simulink model "lab13try1_2024a"  (R2024a)
settings: Solver=VariableStepAuto  StartTime=0.0  StopTime=250  RelTol=1e-3  EnableMultiTasking=on
values from neighbouring files (symbols this model uses):
  CDdatum = CD(1:47,2)    [Presimulink.m]
  CLdatum = CL(1:47,2)    [Presimulink.m]
  Cmdatum = Cm(1:47,2)    [Presimulink.m]
  dCDelev = [dCDn10 dCDn5 dCD0 dCDp5 dCDp10]    [Presimulink.m]
  dCLelev = [dCLn10 dCLn5 dCL0 dCLp5 dCLp10]    [Presimulink.m]
  dCmelev = [dCmn10 dCmn5 dCm0 dCmp5 dCmp10]    [Presimulink.m]
undefined symbols (not defined in the file or in its folder): Cn_datum, Croll_datum, CY_datum, dCn_aileron, dCn_rudder, dCroll_aileron, dCroll_rudder, dCY_aileron, dCY_rudder
libraries: aerolibconvert2 x6, slpidlib x4, aerolibasang x2, shared6dof x1, aerolibadyn x1, aerolibanim x1
settings Model: Creator=davidrwilliams  LastModifiedBy=xan2
settings SolverCC: AlgebraicLoopSolver=TrustRegion
settings DataIOCC: LimitDataPoints=on  ReturnWorkspaceOutputs=off
settings OptimizationCC: ReuseModelBlockBuffer=off  LifeSpan=inf
settings DebuggingCC: UnconnectedInputMsg=warning  UnconnectedOutputMsg=warning  UnconnectedLineMsg=warning  AllowSymbolicDim=off  SFUnexpectedBacktrackingDiag=warning  SFNoUnconditionalDefaultTransitionDiag=warning  SFExecutionAtInitializationDiag=none  ArithmeticOperatorsInVariantConditions=warning
settings ModelReferenceCC: EnableRefExpFcnMdlSchedulingChecks=on  PropagateSignalLabelsOutOfModel=off
settings SFSimCC: SimUseLocalCustomCode=off  CustomCodeUndefinedFunction=UseInterfaceOnly
settings RTWCC: RTWUseLocalCustomCode=off  GPUComputeCapability=3.5
settings CodeAppCC: StateflowObjectComments=on
settings GRTTargetCC: TargetLangStandard=C89/C90 (ANSI)
settings ConfigComp: CovMetricSettings=dw  CovSaveCumulativeToWorkspaceVar=on  CovSaveSingleToWorkspaceVar=on  CovExternalEMLEnable=off  CovBoundaryAbsTol=1.0e-5

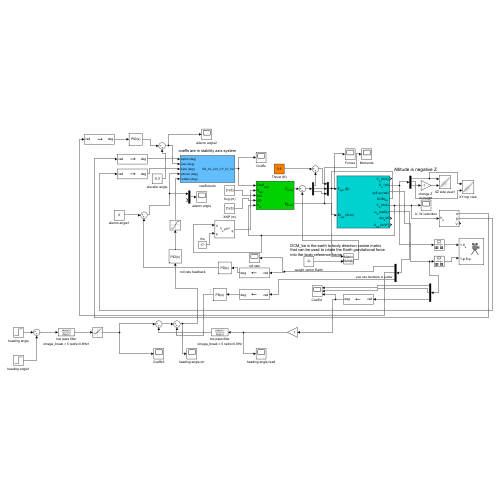
[thumbnail: Simulink's stored preview of the top-level diagram]
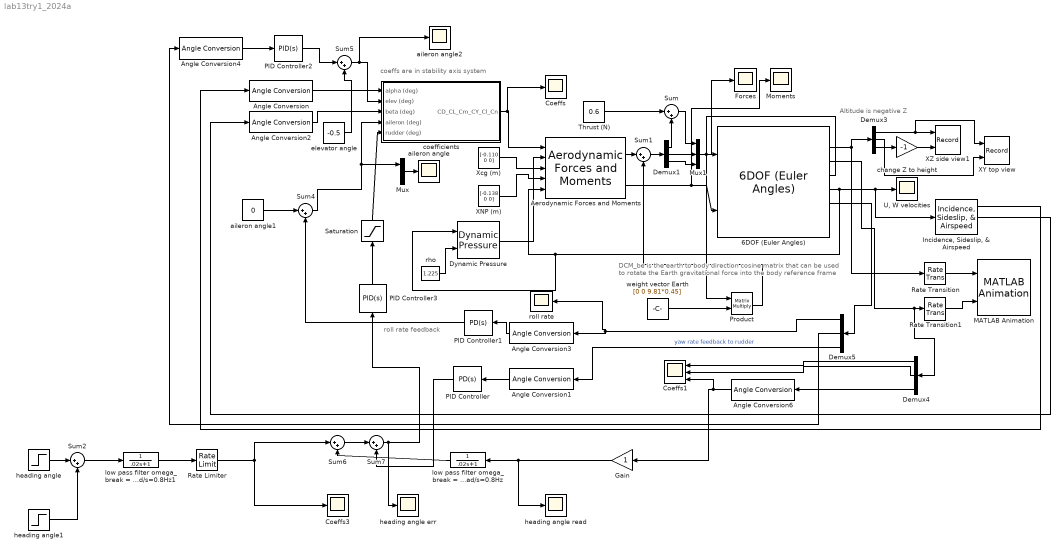
== system lab13try1_2024a ==
  note: roll rate feedback
  note: DCM_be is the earth to body direction cosine matrix
      | that can be used to rotate the Earth gravitational force
      | into the body reference frame
  note: Altitude is negative Z
  note: coeffs are in stability axis system
  6DOF (Euler Angles) : shared6dof/6DOF (Euler Angles)  units=Metric (MKS)  mtype=Fixed  rep=Euler Angles  xme_0=[0 0 -200]  Vm_0=[15 0 2.5]  eul_0=[0 1.4*pi/180 0]  pm_0=[0 0 0]  mass_0=0.45  mass_e=0.5  mass_f=2.0  inertia=[0.00083 0. -0.00118; 0. 0.0428 0.0; -0.00118 0.0 0.0433]  inertia_e=eye(3)  inertia_f=2*eye(3)  k_quat=1.0  vre_flag=on  abi_flag=off  aMode=aMode  xme_statename=''  Vm_statename=''  eul_statename=''  quat_statename=''  pm_statename=''  mass_statename=''
  "Aerodynamic Forces and Moments " : aerolibadyn/Aerodynamic Forces and Moments   inputAxes=Stability  outputForceAxes=Body  outputMomentAxes=Body  S=0.15  b=1  cbar=0.156
  Angle Conversion{,1..4,6} (6 alike) : aerolibconvert2/Angle Conversion  IU=rad  OU=deg
  Coeffs : Scope
  Coeffs1 : Scope  NumInputPorts=3
  Coeffs3 : Scope
  Demux{1,3..5} (4 alike) : Demux  Outputs=3
  Dynamic Pressure : aerolibasang/Dynamic Pressure
  Forces : Scope
  Gain : Gain
  "Incidence, Sideslip, & Airspeed" : aerolibasang/Incidence, Sideslip, & Airspeed
  MATLAB Animation : aerolibanim/MATLAB Animation  Tag=Matlab Animation 6 DOF  Vehicles=1  Geometries='astredwedge.mat'  BoundingBoxCoordinates=[-50,50,-50,50,-50,50]  CameraOffset=[-150,-50,0]  CameraViewAngle=3  SampleTime=0.2  FigurePosition=[8.014000e+02,2.082000e+02,4.480000e+02,3.540000e+02]
  Moments : Scope
  Mux : Mux  Inputs=2
  Mux1 : Mux  Inputs=3
  PID Controller : slpidlib/PID Controller  Controller=PD  Form=Parallel  TimeDomain=Continuous-time  UseExternalTs=off  SampleTime=-1  IntegratorMethod=Forward Euler  FilterMethod=Forward Euler  ControllerParametersSource=internal  P=0.005  I=1  UseKiTs=off  D=0  UseExternalDerivativeSource=off  N=100  UseFilter=on  TunerSelectOption=Transfer Function Based (PID Tuner App)  InitialConditionSource=internal  InitialConditionForIntegrator=0  InitialConditionForFilter=0  DifferentiatorICPrevScaledInput=0  ExternalReset=none  TrackingMode=off  Kt=1  LimitOutput=off  SatLimitsSource=internal  UpperSaturationLimit=inf  LowerSaturationLimit=-inf  LinearizeAsGain=on  AntiWindupMode=none  Kb=1  LimitIntegrator=off  UpperIntegratorSaturationLimit=inf  LowerIntegratorSaturationLimit=-inf  POutMin=[]  POutMax=[]  IOutMin=[]  IOutMax=[]  DOutMin=[]  DOutMax=[]  NOutMin=[]  NOutMax=[]  SumOutMin=[]  SumOutMax=[]  SaturationOutMin=[]  SaturationOutMax=[]  PParamMin=[]  PParamMax=[]  IParamMin=[]  IParamMax=[]  DParamMin=[]  DParamMax=[]  NParamMin=[]  NParamMax=[]  KbParamMin=[]  KbParamMax=[]  KtParamMin=[]  KtParamMax=[]  KbOutMin=[]  KbOutMax=[]  KtOutMin=[]  KtOutMax=[]  IntegratorOutMin=[]  IntegratorOutMax=[]  FilterOutMin=[]  FilterOutMax=[]  SumI1OutMin=[]  SumI1OutMax=[]  SumI2OutMin=[]  SumI2OutMax=[]  SumI3OutMin=[]  SumI3OutMax=[]  SumI4OutMin=[]  SumI4OutMax=[]  SumDOutMin=[]  SumDOutMax=[]  DifferentiatorOutMin=[]  DifferentiatorOutMax=[]  FilterDiffOutCoefMin=[]  FilterDiffOutCoefMax=[]  ReciprocalOutMin=[]  ReciprocalOutMax=[]  SumDenOutMin=[]  SumDenOutMax=[]  SumNumOutMin=[]  SumNumOutMax=[]  DivideOutMin=[]  DivideOutMax=[]  UdiffTsProdOutMin=[]  UdiffTsProdOutMax=[]  NTsProdOutMin=[]  NTsProdOutMax=[]  UintegralTsProdOutMin=[]  UintegralTsProdOutMax=[]  UngainTsProdOutMin=[]  UngainTsProdOutMax=[]  ClampingZeroOutDataTypeStr=Inherit: Inherit via back propagation  ClampingZeroOutMin=[]  ClampingZeroOutMax=[]  FilterDenConstantOutDataTypeStr=Inherit: Inherit via back propagation  FilterDenConstantOutMin=[]  FilterDenConstantOutMax=[]  PCopyOutDataTypeStr=Inherit: Inherit via back propagation  PCopyOutMin=[]  PCopyOutMax=[]  NCopyOutDataTypeStr=Inherit: Inherit via back propagation  NCopyOutMin=[]  NCopyOutMax=[]  IntegratorContinuousStateAttributes=''  IntegratorStateMustResolveToSignalObject=off  IntegratorRTWStateStorageClass=Auto  FilterContinuousStateAttributes=''  FilterStateMustResolveToSignalObject=off  FilterRTWStateStorageClass=Auto  ParallelPVariant=InternalParameters  IdealPVariant=Disabled  IVariant=Disabled  DVariant=InternalParameters  IntegratorVariant=Disabled  SatVariant=Disabled  AWVariant=Disabled  PCopyVariant=Disabled  TRVariant=Disabled  FdbkBlocksVariant=Forward  IdealPFdbkVariant=Disabled  SatFdbkVariant=Disabled  DerivativeFilterVariant=ContFilter  NVariant=InternalParameters  NCopyVariant=Disabled  FilterICVariant=InternalICsFilter  IntegratorICVariant=Disabled  ExternalResetVariant=Disabled  TRSumVariant=Passthrough  SumFdbkVariant=Disabled  SumVariant=Sum_PD  TsampFilterVariant=InternalTs  TsampNgainVariant=Passthrough  TsampIntegralVariant=Disabled_SignalSpec  ExternalSaturationOutDataTypeStr=Inherit: Same as second input  DerivativeSourceVariant=ErrorSignal
  PID Controller1 : slpidlib/PID Controller  Controller=PD  Form=Parallel  TimeDomain=Continuous-time  UseExternalTs=off  SampleTime=-1  IntegratorMethod=Forward Euler  FilterMethod=Forward Euler  ControllerParametersSource=internal  P=-0.5  I=1  UseKiTs=off  D=0  UseExternalDerivativeSource=off  N=100  UseFilter=on  TunerSelectOption=Transfer Function Based (PID Tuner App)  InitialConditionSource=internal  InitialConditionForIntegrator=0  InitialConditionForFilter=0  DifferentiatorICPrevScaledInput=0  ExternalReset=none  TrackingMode=off  Kt=1  LimitOutput=off  SatLimitsSource=internal  UpperSaturationLimit=inf  LowerSaturationLimit=-inf  LinearizeAsGain=on  AntiWindupMode=none  Kb=1  LimitIntegrator=off  UpperIntegratorSaturationLimit=inf  LowerIntegratorSaturationLimit=-inf  POutMin=[]  POutMax=[]  IOutMin=[]  IOutMax=[]  DOutMin=[]  DOutMax=[]  NOutMin=[]  NOutMax=[]  SumOutMin=[]  SumOutMax=[]  SaturationOutMin=[]  SaturationOutMax=[]  PParamMin=[]  PParamMax=[]  IParamMin=[]  IParamMax=[]  DParamMin=[]  DParamMax=[]  NParamMin=[]  NParamMax=[]  KbParamMin=[]  KbParamMax=[]  KtParamMin=[]  KtParamMax=[]  KbOutMin=[]  KbOutMax=[]  KtOutMin=[]  KtOutMax=[]  IntegratorOutMin=[]  IntegratorOutMax=[]  FilterOutMin=[]  FilterOutMax=[]  SumI1OutMin=[]  SumI1OutMax=[]  SumI2OutMin=[]  SumI2OutMax=[]  SumI3OutMin=[]  SumI3OutMax=[]  SumI4OutMin=[]  SumI4OutMax=[]  SumDOutMin=[]  SumDOutMax=[]  DifferentiatorOutMin=[]  DifferentiatorOutMax=[]  FilterDiffOutCoefMin=[]  FilterDiffOutCoefMax=[]  ReciprocalOutMin=[]  ReciprocalOutMax=[]  SumDenOutMin=[]  SumDenOutMax=[]  SumNumOutMin=[]  SumNumOutMax=[]  DivideOutMin=[]  DivideOutMax=[]  UdiffTsProdOutMin=[]  UdiffTsProdOutMax=[]  NTsProdOutMin=[]  NTsProdOutMax=[]  UintegralTsProdOutMin=[]  UintegralTsProdOutMax=[]  UngainTsProdOutMin=[]  UngainTsProdOutMax=[]  ClampingZeroOutDataTypeStr=Inherit: Inherit via back propagation  ClampingZeroOutMin=[]  ClampingZeroOutMax=[]  FilterDenConstantOutDataTypeStr=Inherit: Inherit via back propagation  FilterDenConstantOutMin=[]  FilterDenConstantOutMax=[]  PCopyOutDataTypeStr=Inherit: Inherit via back propagation  PCopyOutMin=[]  PCopyOutMax=[]  NCopyOutDataTypeStr=Inherit: Inherit via back propagation  NCopyOutMin=[]  NCopyOutMax=[]  IntegratorContinuousStateAttributes=''  IntegratorStateMustResolveToSignalObject=off  IntegratorRTWStateStorageClass=Auto  FilterContinuousStateAttributes=''  FilterStateMustResolveToSignalObject=off  FilterRTWStateStorageClass=Auto  ParallelPVariant=InternalParameters  IdealPVariant=Disabled  IVariant=Disabled  DVariant=InternalParameters  IntegratorVariant=Disabled  SatVariant=Disabled  AWVariant=Disabled  PCopyVariant=Disabled  TRVariant=Disabled  FdbkBlocksVariant=Forward  IdealPFdbkVariant=Disabled  SatFdbkVariant=Disabled  DerivativeFilterVariant=ContFilter  NVariant=InternalParameters  NCopyVariant=Disabled  FilterICVariant=InternalICsFilter  IntegratorICVariant=Disabled  ExternalResetVariant=Disabled  TRSumVariant=Passthrough  SumFdbkVariant=Disabled  SumVariant=Sum_PD  TsampFilterVariant=InternalTs  TsampNgainVariant=Passthrough  TsampIntegralVariant=Disabled_SignalSpec  ExternalSaturationOutDataTypeStr=Inherit: Same as second input  DerivativeSourceVariant=ErrorSignal
  PID Controller2 : slpidlib/PID Controller  Controller=PID  Form=Parallel  TimeDomain=Continuous-time  UseExternalTs=off  SampleTime=-1  IntegratorMethod=Forward Euler  FilterMethod=Forward Euler  ControllerParametersSource=internal  P=1  I=0  UseKiTs=off  D=0  UseExternalDerivativeSource=off  N=100  UseFilter=on  TunerSelectOption=Transfer Function Based (PID Tuner App)  InitialConditionSource=internal  InitialConditionForIntegrator=0  InitialConditionForFilter=0  DifferentiatorICPrevScaledInput=0  ExternalReset=none  TrackingMode=off  Kt=1  LimitOutput=off  SatLimitsSource=internal  UpperSaturationLimit=inf  LowerSaturationLimit=-inf  LinearizeAsGain=on  AntiWindupMode=none  Kb=1  LimitIntegrator=off  UpperIntegratorSaturationLimit=inf  LowerIntegratorSaturationLimit=-inf  POutMin=[]  POutMax=[]  IOutMin=[]  IOutMax=[]  DOutMin=[]  DOutMax=[]  NOutMin=[]  NOutMax=[]  SumOutMin=[]  SumOutMax=[]  SaturationOutMin=[]  SaturationOutMax=[]  PParamMin=[]  PParamMax=[]  IParamMin=[]  IParamMax=[]  DParamMin=[]  DParamMax=[]  NParamMin=[]  NParamMax=[]  KbParamMin=[]  KbParamMax=[]  KtParamMin=[]  KtParamMax=[]  KbOutMin=[]  KbOutMax=[]  KtOutMin=[]  KtOutMax=[]  IntegratorOutMin=[]  IntegratorOutMax=[]  FilterOutMin=[]  FilterOutMax=[]  SumI1OutMin=[]  SumI1OutMax=[]  SumI2OutMin=[]  SumI2OutMax=[]  SumI3OutMin=[]  SumI3OutMax=[]  SumI4OutMin=[]  SumI4OutMax=[]  SumDOutMin=[]  SumDOutMax=[]  DifferentiatorOutMin=[]  DifferentiatorOutMax=[]  FilterDiffOutCoefMin=[]  FilterDiffOutCoefMax=[]  ReciprocalOutMin=[]  ReciprocalOutMax=[]  SumDenOutMin=[]  SumDenOutMax=[]  SumNumOutMin=[]  SumNumOutMax=[]  DivideOutMin=[]  DivideOutMax=[]  UdiffTsProdOutMin=[]  UdiffTsProdOutMax=[]  NTsProdOutMin=[]  NTsProdOutMax=[]  UintegralTsProdOutMin=[]  UintegralTsProdOutMax=[]  UngainTsProdOutMin=[]  UngainTsProdOutMax=[]  ClampingZeroOutDataTypeStr=Inherit: Inherit via back propagation  ClampingZeroOutMin=[]  ClampingZeroOutMax=[]  FilterDenConstantOutDataTypeStr=Inherit: Inherit via back propagation  FilterDenConstantOutMin=[]  FilterDenConstantOutMax=[]  PCopyOutDataTypeStr=Inherit: Inherit via back propagation  PCopyOutMin=[]  PCopyOutMax=[]  NCopyOutDataTypeStr=Inherit: Inherit via back propagation  NCopyOutMin=[]  NCopyOutMax=[]  IntegratorContinuousStateAttributes=''  IntegratorStateMustResolveToSignalObject=off  IntegratorRTWStateStorageClass=Auto  FilterContinuousStateAttributes=''  FilterStateMustResolveToSignalObject=off  FilterRTWStateStorageClass=Auto  ParallelPVariant=InternalParameters  IdealPVariant=Disabled  IVariant=InternalParameters  DVariant=InternalParameters  IntegratorVariant=Continuous  SatVariant=Disabled  AWVariant=Passthrough  PCopyVariant=Disabled  TRVariant=Disabled  FdbkBlocksVariant=Forward  IdealPFdbkVariant=Disabled  SatFdbkVariant=Disabled  DerivativeFilterVariant=ContFilter  NVariant=InternalParameters  NCopyVariant=Disabled  FilterICVariant=InternalICsFilter  IntegratorICVariant=InternalICs  ExternalResetVariant=Disabled  TRSumVariant=Passthrough  SumFdbkVariant=Disabled  SumVariant=Sum_PID  TsampFilterVariant=InternalTs  TsampNgainVariant=Passthrough  TsampIntegralVariant=Disabled_SignalSpec  ExternalSaturationOutDataTypeStr=Inherit: Same as second input  DerivativeSourceVariant=ErrorSignal
  PID Controller3 : slpidlib/PID Controller  Controller=PID  Form=Parallel  TimeDomain=Continuous-time  UseExternalTs=off  SampleTime=-1  IntegratorMethod=Forward Euler  FilterMethod=Forward Euler  ControllerParametersSource=internal  P=1  I=0  UseKiTs=off  D=0.3  UseExternalDerivativeSource=off  N=100  UseFilter=on  TunerSelectOption=Transfer Function Based (PID Tuner App)  InitialConditionSource=internal  InitialConditionForIntegrator=0  InitialConditionForFilter=0  DifferentiatorICPrevScaledInput=0  ExternalReset=none  TrackingMode=off  Kt=1  LimitOutput=off  SatLimitsSource=internal  UpperSaturationLimit=inf  LowerSaturationLimit=-inf  LinearizeAsGain=on  AntiWindupMode=none  Kb=1  LimitIntegrator=off  UpperIntegratorSaturationLimit=inf  LowerIntegratorSaturationLimit=-inf  POutMin=[]  POutMax=[]  IOutMin=[]  IOutMax=[]  DOutMin=[]  DOutMax=[]  NOutMin=[]  NOutMax=[]  SumOutMin=[]  SumOutMax=[]  SaturationOutMin=[]  SaturationOutMax=[]  PParamMin=[]  PParamMax=[]  IParamMin=[]  IParamMax=[]  DParamMin=[]  DParamMax=[]  NParamMin=[]  NParamMax=[]  KbParamMin=[]  KbParamMax=[]  KtParamMin=[]  KtParamMax=[]  KbOutMin=[]  KbOutMax=[]  KtOutMin=[]  KtOutMax=[]  IntegratorOutMin=[]  IntegratorOutMax=[]  FilterOutMin=[]  FilterOutMax=[]  SumI1OutMin=[]  SumI1OutMax=[]  SumI2OutMin=[]  SumI2OutMax=[]  SumI3OutMin=[]  SumI3OutMax=[]  SumI4OutMin=[]  SumI4OutMax=[]  SumDOutMin=[]  SumDOutMax=[]  DifferentiatorOutMin=[]  DifferentiatorOutMax=[]  FilterDiffOutCoefMin=[]  FilterDiffOutCoefMax=[]  ReciprocalOutMin=[]  ReciprocalOutMax=[]  SumDenOutMin=[]  SumDenOutMax=[]  SumNumOutMin=[]  SumNumOutMax=[]  DivideOutMin=[]  DivideOutMax=[]  UdiffTsProdOutMin=[]  UdiffTsProdOutMax=[]  NTsProdOutMin=[]  NTsProdOutMax=[]  UintegralTsProdOutMin=[]  UintegralTsProdOutMax=[]  UngainTsProdOutMin=[]  UngainTsProdOutMax=[]  ClampingZeroOutDataTypeStr=Inherit: Inherit via back propagation  ClampingZeroOutMin=[]  ClampingZeroOutMax=[]  FilterDenConstantOutDataTypeStr=Inherit: Inherit via back propagation  FilterDenConstantOutMin=[]  FilterDenConstantOutMax=[]  PCopyOutDataTypeStr=Inherit: Inherit via back propagation  PCopyOutMin=[]  PCopyOutMax=[]  NCopyOutDataTypeStr=Inherit: Inherit via back propagation  NCopyOutMin=[]  NCopyOutMax=[]  IntegratorContinuousStateAttributes=''  IntegratorStateMustResolveToSignalObject=off  IntegratorRTWStateStorageClass=Auto  FilterContinuousStateAttributes=''  FilterStateMustResolveToSignalObject=off  FilterRTWStateStorageClass=Auto  ParallelPVariant=InternalParameters  IdealPVariant=Disabled  IVariant=InternalParameters  DVariant=InternalParameters  IntegratorVariant=Continuous  SatVariant=Disabled  AWVariant=Passthrough  PCopyVariant=Disabled  TRVariant=Disabled  FdbkBlocksVariant=Forward  IdealPFdbkVariant=Disabled  SatFdbkVariant=Disabled  DerivativeFilterVariant=ContFilter  NVariant=InternalParameters  NCopyVariant=Disabled  FilterICVariant=InternalICsFilter  IntegratorICVariant=InternalICs  ExternalResetVariant=Disabled  TRSumVariant=Passthrough  SumFdbkVariant=Disabled  SumVariant=Sum_PID  TsampFilterVariant=InternalTs  TsampNgainVariant=Passthrough  TsampIntegralVariant=Disabled_SignalSpec  ExternalSaturationOutDataTypeStr=Inherit: Same as second input  DerivativeSourceVariant=ErrorSignal
  Product : Product  Multiplication=Matrix(*)
  Rate Limiter : RateLimiter  RisingSlewLimit=10  FallingSlewLimit=-10  SampleTimeMode=inherited
  Rate Transition : RateTransition
  Rate Transition1 : RateTransition
  Saturation : Saturate  UpperLimit=10  LowerLimit=-10
  Sum{,1..2,4..7} (7 alike) : Sum  Inputs=|++
  Thrust (N) : Constant  Value=0.6
  "U, W velocities" : Scope
  XNP (m) : Constant  Value=[-0.138 0 0]
  XY top view : Record  FileSettingsInternal="{\"entries\":[{\"content\":{\"excelSettings\":{\"content\":{},\"type\":\"Streamout.ExcelSettings\"},\"parquetSettings\":{\"content\":{},\"type\":\"Streamout.ParquetSettings\"}},\"type\":\"Streamout.FileSettingStorage\",\"uuid\":\"\"}],\"packageUris\":[\"http:\\/\\/schema.mathworks.com\\/mf0\\/streamout_blocks\\/R2020a\"],\"version\":\"1.0\"}"  Layout=[1 1]  SignalsInternal="{\"entries\":[{\"content\":{\"signals\":[{\"content\":{\"blockPath\":[],\"dimensions\":[1],\"domain\":\"\",\"lineColor\":\"#a2142f\",\"plots\":[ 1 ],\"port\":1,\"signalID\":1,\"signalName\":\"Demux3:1\"},\"type\":\"RecordBlkView.Signal\",\"uuid\":\"\"},{\"content\":{\"blockPath\":[],\"dimensions\":[1],\"domain\":\"\",\"lineColor\":\"#139fff\",\"plots\":[ 1 ],\"port\":2,\"signalID\":2,\"signalName\":\"Demux3:2\"},\"type\":\"RecordBlkView.Signal\",\"uuid\":\"\"}]},\"type\":\"RecordBlkView.InputSignals\",\"uuid\":\"\"}],\"packageUris\":[\"http:\\/\\/schema.mathworks.com\\/mf0\\/streamout_blocks\\/R2020a\"],\"version\":\"1.0\"}"  VisualizationBindings="{\"xyplotplugin\":{\"info\":[{\"series\":[{\"bindingParametersList\":[{\"parameter\":\"X-Axis\",\"signalID\":1,\"signalName\":\"Demux3:1\"},{\"parameter\":\"Y-Axis\",\"signalID\":2,\"signalName\":\"Demux3:2\"}],\"seriesID\":0}],\"subplotID\":1}]}}"  CompatibilityTag=XY  st=-1
  XZ side view1 : Record  FileSettingsInternal="{\"entries\":[{\"content\":{\"excelSettings\":{\"content\":{},\"type\":\"Streamout.ExcelSettings\"},\"parquetSettings\":{\"content\":{},\"type\":\"Streamout.ParquetSettings\"}},\"type\":\"Streamout.FileSettingStorage\",\"uuid\":\"\"}],\"packageUris\":[\"http:\\/\\/schema.mathworks.com\\/mf0\\/streamout_blocks\\/R2020a\"],\"version\":\"1.0\"}"  Layout=[1 1]  SignalsInternal="{\"entries\":[{\"content\":{\"signals\":[{\"content\":{\"blockPath\":[],\"dimensions\":[1],\"domain\":\"\",\"lineColor\":\"#a2142f\",\"plots\":[ 1 ],\"port\":1,\"signalID\":1,\"signalName\":\"Demux3:1\"},\"type\":\"RecordBlkView.Signal\",\"uuid\":\"\"},{\"content\":{\"blockPath\":[],\"dimensions\":[1],\"domain\":\"\",\"lineColor\":\"#139fff\",\"plots\":[ 1 ],\"port\":2,\"signalID\":2,\"signalName\":\"change Z \\nto height\"},\"type\":\"RecordBlkView.Signal\",\"uuid\":\"\"}]},\"type\":\"RecordBlkView.InputSignals\",\"uuid\":\"\"}],\"packageUris\":[\"http:\\/\\/schema.mathworks.com\\/mf0\\/streamout_blocks\\/R2020a\"],\"version\":\"1.0\"}"  VisualizationBindings="{\"xyplotplugin\":{\"info\":[{\"series\":[{\"bindingParametersList\":[{\"parameter\":\"X-Axis\",\"signalID\":1,\"signalName\":\"Demux3:1\"},{\"parameter\":\"Y-Axis\",\"signalID\":2,\"signalName\":\"change Z \\nto height\"}],\"seriesID\":0}],\"subplotID\":1}]}}"  CompatibilityTag=XY  st=-1
  Xcg (m) : Constant  Value=[-0.110 0 0]
  aileron angle : Scope
  aileron angle1 : Constant  Value=0
  aileron angle2 : Scope
  change Z to height : Gain  Gain=-1
  coefficients : Subsystem
  elevator angle : Constant  Value=-0.5
  heading angle : Step  Time=50  After=90
  heading angle err : Scope
  heading angle read : Scope
  heading angle1 : Step  Time=200  After=80
  low pass filter omega_break = 5 rad/s=0.8Hz : TransferFcn  Denominator=[.02 1]
  low pass filter omega_break = 5 rad/s=0.8Hz1 : TransferFcn  Denominator=[.02 1]
  rho : Constant  Value=1.225
  roll rate : Scope
  weight vector Earth : Constant  Value=[0 0 9.81*0.45]
  wires:
  rho/1 -> Dynamic Pressure/2
  Dynamic Pressure/1 -> "Aerodynamic Forces and Moments "/2
  Demux1/3 -> Mux1/3
  Demux1/2 -> Mux1/2
  Xcg (m)/1 -> "Aerodynamic Forces and Moments "/3
  XNP (m)/1 -> "Aerodynamic Forces and Moments "/4
  coefficients/1(CD_CL_Cm_CY_Cl_Cn) -> Coeffs/1, "Aerodynamic Forces and Moments "/1
  6DOF (Euler Angles)/2 -> Demux3/1, Rate Transition/1
  Demux3/1 -> XZ side view1/1, XY top view/1
  Sum/1 -> Mux1/1
  Angle Conversion/1 -> coefficients/1(alpha (deg))
  Mux1/1 -> Forces/1, 6DOF (Euler Angles)/1
  "Aerodynamic Forces and Moments "/2 -> Moments/1, 6DOF (Euler Angles)/2
  Demux3/3 -> change Z to height/1
  weight vector Earth/1 -> Product/2
  Product/1 -> Sum1/2
  6DOF (Euler Angles)/4 -> Product/1
  "Aerodynamic Forces and Moments "/1 -> Sum1/1
  Sum1/1 -> Demux1/1
  Demux3/2 -> XY top view/2
  6DOF (Euler Angles)/6 -> Demux5/1
  Angle Conversion1/1 -> PID Controller/1
  Demux5/1 -> roll rate/1, Angle Conversion3/1
  Rate Transition/1 -> MATLAB Animation/1
  Rate Transition1/1 -> MATLAB Animation/2
  Demux5/2 -> Angle Conversion4/1
  6DOF (Euler Angles)/5 -> "Incidence, Sideslip, & Airspeed"/1, "U, W velocities"/1, Dynamic Pressure/1, "Aerodynamic Forces and Moments "/5
  "Incidence, Sideslip, & Airspeed"/1 -> Angle Conversion/1
  Angle Conversion2/1 -> coefficients/3(beta (deg))
  "Incidence, Sideslip, & Airspeed"/2 -> Angle Conversion2/1
  Angle Conversion3/1 -> PID Controller1/1
  Mux/1 -> aileron angle/1
  PID Controller/1 -> Sum7/2
  PID Controller1/1 -> Sum4/2
  Demux5/3 -> Angle Conversion1/1  "yaw rate feedback to rudder"
  PID Controller2/1 -> Sum5/1
  Angle Conversion4/1 -> PID Controller2/1
  elevator angle/1 -> Sum5/2
  aileron angle1/1 -> Sum4/1
  change Z to height/1 -> XZ side view1/2
  Sum6/1 -> Sum7/1
  low pass filter omega_break = 5 rad/s=0.8Hz/1 -> Sum6/2
  Sum4/1 -> coefficients/4(aileron (deg)), Mux/1
  Demux4/1 -> Coeffs1/1
  Demux4/2 -> Coeffs1/2
  Sum5/1 -> aileron angle2/1, coefficients/2(elev (deg))
  Saturation/1 -> coefficients/5(rudder (deg))
  Sum7/1 -> heading angle err/1, PID Controller3/1
  PID Controller3/1 -> Saturation/1
  Rate Limiter/1 -> Sum6/1, Coeffs3/1
  low pass filter omega_break = 5 rad/s=0.8Hz1/1 -> Rate Limiter/1
  heading angle/1 -> Sum2/1
  Demux1/1 -> Sum/2
  Thrust (N)/1 -> Sum/1
  Sum2/1 -> low pass filter omega_break = 5 rad/s=0.8Hz1/1
  heading angle1/1 -> Sum2/2
  Gain/1 -> heading angle read/1, low pass filter omega_break = 5 rad/s=0.8Hz/1
  6DOF (Euler Angles)/3 -> Demux4/1, Rate Transition1/1
  Demux4/3 -> Angle Conversion6/1
  Angle Conversion6/1 -> Gain/1, Coeffs1/3

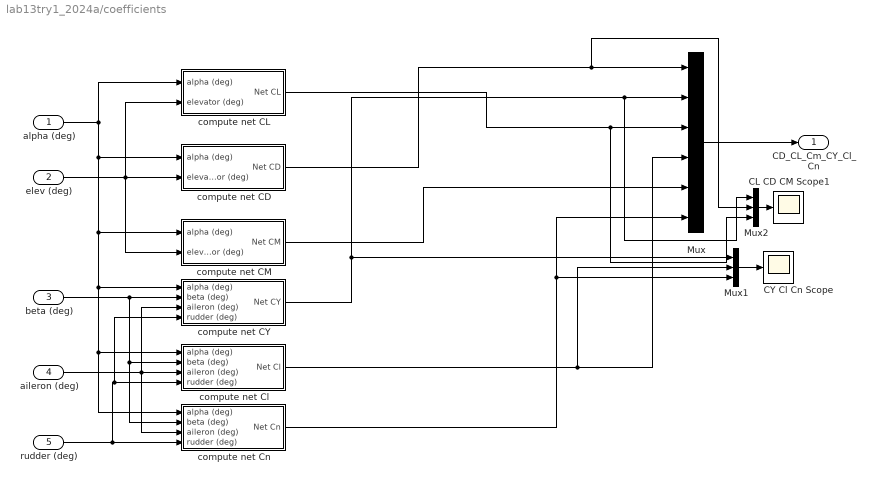
== system lab13try1_2024a/coefficients ==
  alpha (deg) : Inport
  elev (deg) : Inport  Port=2
  beta (deg) : Inport  Port=3
  aileron (deg) : Inport  Port=4
  rudder (deg) : Inport  Port=5
  CL CD CM Scope1 : Scope
  CY Cl Cn Scope : Scope
  Mux : Mux  Inputs=6
  Mux1 : Mux  Inputs=3
  Mux2 : Mux  Inputs=3
  compute net CD : Subsystem
  compute net CL : Subsystem
  compute net CM : Subsystem
  compute net CY : Subsystem
  compute net Cl : Subsystem
  compute net Cn : Subsystem
  CD_CL_Cm_CY_Cl_Cn : Outport  VectorParamsAs1DForOutWhenUnconnected=off
  wires:
  compute net Cn/1(Net Cn) -> Mux1/3, Mux/6
  Mux/1 -> CD_CL_Cm_CY_Cl_Cn/1
  elev (deg)/1 -> compute net CD/2(elevator (deg)), compute net CM/2(elevator (deg)), compute net CL/2(elevator (deg))
  alpha (deg)/1 -> compute net CD/1(alpha (deg)), compute net Cn/1(alpha (deg)), compute net Cl/1(alpha (deg)), compute net CY/1(alpha (deg)), compute net CM/1(alpha (deg)), compute net CL/1(alpha (deg))
  compute net CD/1(Net CD) -> Mux2/2, Mux/1
  compute net CL/1(Net CL) -> Mux2/3, Mux/3
  compute net CM/1(Net CM) -> Mux/5
  compute net Cl/1(Net Cl) -> Mux1/2, Mux/4
  compute net CY/1(Net CY) -> Mux1/1, Mux2/1, Mux/2
  aileron (deg)/1 -> compute net Cl/3(aileron (deg)), compute net CY/3(aileron (deg)), compute net Cn/3(aileron (deg))
  beta (deg)/1 -> compute net Cn/2(beta (deg)), compute net Cl/2(beta (deg)), compute net CY/2(beta (deg))
  rudder (deg)/1 -> compute net CY/4(rudder (deg)), compute net Cl/4(rudder (deg)), compute net Cn/4(rudder (deg))
  Mux1/1 -> CY Cl Cn Scope/1
  Mux2/1 -> CL CD CM Scope1/1

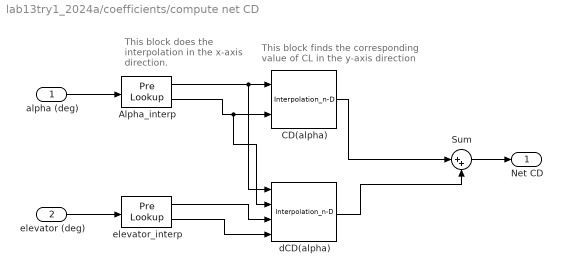
== system lab13try1_2024a/coefficients/compute net CD ==
  note: This block finds the corresponding
      | value of CL in the y-axis direction
  note: This block does the interpolation in the
      | x-axis direction.
  alpha (deg) : Inport
  elevator (deg) : Inport  Port=2
  Alpha_interp : PreLookup  BreakpointsData=alpha  BeginIndexSearchUsingPreviousIndexResult=on  ExtrapMethod=Linear
  CD(alpha) : Interpolation_n-D  NumberOfTableDimensions=1  Table=CDdatum  RemoveProtectionIndex=on
      settings: InputPortMap=u0,u1
  Sum : Sum  Inputs=|++
  dCD(alpha) : Interpolation_n-D  Table=dCDelev
  elevator_interp : PreLookup  BreakpointsData=delev  BeginIndexSearchUsingPreviousIndexResult=on  ExtrapMethod=Linear
  Net CD : Outport  VectorParamsAs1DForOutWhenUnconnected=off
  wires:
  Alpha_interp/1 -> dCD(alpha)/1, CD(alpha)/1
  Alpha_interp/2 -> dCD(alpha)/2, CD(alpha)/2
  CD(alpha)/1 -> Sum/1
  alpha (deg)/1 -> Alpha_interp/1
  elevator (deg)/1 -> elevator_interp/1
  elevator_interp/2 -> dCD(alpha)/4
  elevator_interp/1 -> dCD(alpha)/3
  dCD(alpha)/1 -> Sum/2
  Sum/1 -> Net CD/1

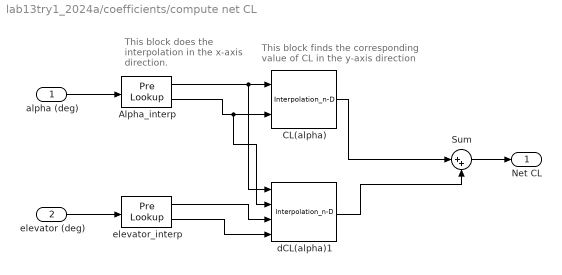
== system lab13try1_2024a/coefficients/compute net CL ==
  note: This block finds the corresponding
      | value of CL in the y-axis direction
  note: This block does the interpolation in the
      | x-axis direction.
  alpha (deg) : Inport
  elevator (deg) : Inport  Port=2
  Alpha_interp : PreLookup  BreakpointsData=alpha  BeginIndexSearchUsingPreviousIndexResult=on  ExtrapMethod=Linear
  CL(alpha) : Interpolation_n-D  NumberOfTableDimensions=1  Table=CLdatum  RemoveProtectionIndex=on
      settings: InputPortMap=u0,u1
  Sum : Sum  Inputs=|++
  dCL(alpha)1 : Interpolation_n-D  Table=dCLelev
  elevator_interp : PreLookup  BreakpointsData=delev  BeginIndexSearchUsingPreviousIndexResult=on  ExtrapMethod=Linear
  Net CL : Outport  VectorParamsAs1DForOutWhenUnconnected=off
  wires:
  Alpha_interp/1 -> dCL(alpha)1/1, CL(alpha)/1
  Alpha_interp/2 -> dCL(alpha)1/2, CL(alpha)/2
  CL(alpha)/1 -> Sum/1
  alpha (deg)/1 -> Alpha_interp/1
  elevator (deg)/1 -> elevator_interp/1
  elevator_interp/2 -> dCL(alpha)1/4
  elevator_interp/1 -> dCL(alpha)1/3
  dCL(alpha)1/1 -> Sum/2
  Sum/1 -> Net CL/1

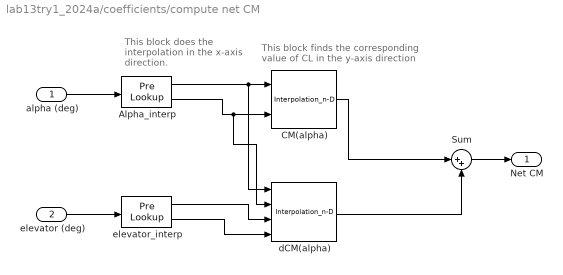
== system lab13try1_2024a/coefficients/compute net CM ==
  note: This block finds the corresponding
      | value of CL in the y-axis direction
  note: This block does the interpolation in the
      | x-axis direction.
  alpha (deg) : Inport
  elevator (deg) : Inport  Port=2
  Alpha_interp : PreLookup  BreakpointsData=alpha  BeginIndexSearchUsingPreviousIndexResult=on  ExtrapMethod=Linear
  CM(alpha) : Interpolation_n-D  NumberOfTableDimensions=1  Table=Cmdatum  RemoveProtectionIndex=on
      settings: InputPortMap=u0,u1
  Sum : Sum  Inputs=|++
  dCM(alpha) : Interpolation_n-D  Table=dCmelev
  elevator_interp : PreLookup  BreakpointsData=delev  BeginIndexSearchUsingPreviousIndexResult=on  ExtrapMethod=Linear
  Net CM : Outport  VectorParamsAs1DForOutWhenUnconnected=off
  wires:
  Alpha_interp/1 -> dCM(alpha)/1, CM(alpha)/1
  Alpha_interp/2 -> dCM(alpha)/2, CM(alpha)/2
  CM(alpha)/1 -> Sum/1
  alpha (deg)/1 -> Alpha_interp/1
  elevator (deg)/1 -> elevator_interp/1
  elevator_interp/2 -> dCM(alpha)/4
  elevator_interp/1 -> dCM(alpha)/3
  Sum/1 -> Net CM/1
  dCM(alpha)/1 -> Sum/2

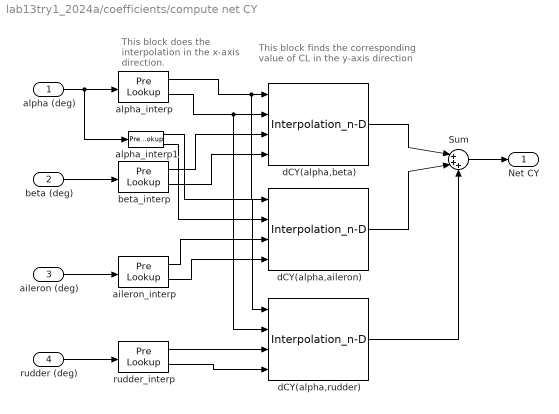
== system lab13try1_2024a/coefficients/compute net CY ==
  note: This block finds the corresponding
      | value of CL in the y-axis direction
  note: This block does the interpolation in the
      | x-axis direction.
  alpha (deg) : Inport
  beta (deg) : Inport  Port=2
  aileron (deg) : Inport  Port=3
  rudder (deg) : Inport  Port=4
  Sum : Sum  Inputs=|+++
  aileron_interp : PreLookup  BreakpointsData=aileron  BeginIndexSearchUsingPreviousIndexResult=on  ExtrapMethod=Linear
  alpha_interp : PreLookup  BreakpointsData=alphalatrud  BeginIndexSearchUsingPreviousIndexResult=on  ExtrapMethod=Linear
  alpha_interp1 : PreLookup  BreakpointsData=alphaaileron  BeginIndexSearchUsingPreviousIndexResult=on  ExtrapMethod=Linear
  beta_interp : PreLookup  BreakpointsData=beta  BeginIndexSearchUsingPreviousIndexResult=on  ExtrapMethod=Linear
  dCY(alpha,aileron) : Interpolation_n-D  Table=dCY_aileron
  dCY(alpha,beta) : Interpolation_n-D  Table=CY_datum
  dCY(alpha,rudder) : Interpolation_n-D  Table=dCY_rudder
  rudder_interp : PreLookup  BreakpointsData=rudder  BeginIndexSearchUsingPreviousIndexResult=on  ExtrapMethod=Linear
  Net CY : Outport  VectorParamsAs1DForOutWhenUnconnected=off
  wires:
  beta (deg)/1 -> beta_interp/1
  Sum/1 -> Net CY/1
  aileron (deg)/1 -> aileron_interp/1
  rudder (deg)/1 -> rudder_interp/1
  beta_interp/1 -> dCY(alpha,beta)/3
  beta_interp/2 -> dCY(alpha,beta)/4
  rudder_interp/2 -> dCY(alpha,rudder)/4
  aileron_interp/1 -> dCY(alpha,aileron)/3
  aileron_interp/2 -> dCY(alpha,aileron)/4
  rudder_interp/1 -> dCY(alpha,rudder)/3
  alpha (deg)/1 -> alpha_interp1/1, alpha_interp/1
  alpha_interp/2 -> dCY(alpha,rudder)/2, dCY(alpha,beta)/2
  alpha_interp/1 -> dCY(alpha,rudder)/1, dCY(alpha,beta)/1
  dCY(alpha,aileron)/1 -> Sum/2
  dCY(alpha,beta)/1 -> Sum/1
  alpha_interp1/1 -> dCY(alpha,aileron)/1
  alpha_interp1/2 -> dCY(alpha,aileron)/2
  dCY(alpha,rudder)/1 -> Sum/3

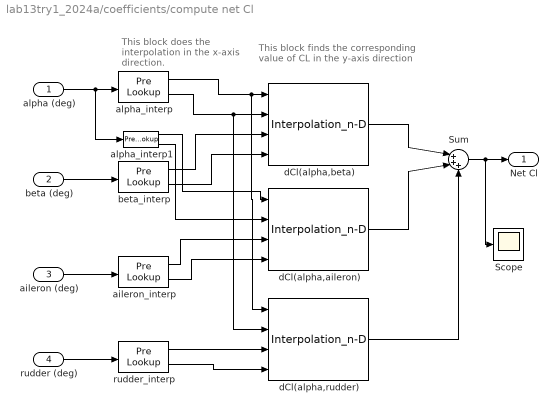
== system lab13try1_2024a/coefficients/compute net Cl ==
  note: This block finds the corresponding
      | value of CL in the y-axis direction
  note: This block does the interpolation in the
      | x-axis direction.
  alpha (deg) : Inport
  beta (deg) : Inport  Port=2
  aileron (deg) : Inport  Port=3
  rudder (deg) : Inport  Port=4
  Scope : Scope
  Sum : Sum  Inputs=|+++
  aileron_interp : PreLookup  BreakpointsData=aileron  BeginIndexSearchUsingPreviousIndexResult=on  ExtrapMethod=Linear
  alpha_interp : PreLookup  BreakpointsData=alphalatrud  BeginIndexSearchUsingPreviousIndexResult=on  ExtrapMethod=Linear
  alpha_interp1 : PreLookup  BreakpointsData=alphaaileron  BeginIndexSearchUsingPreviousIndexResult=on  ExtrapMethod=Linear
  beta_interp : PreLookup  BreakpointsData=beta  BeginIndexSearchUsingPreviousIndexResult=on  ExtrapMethod=Linear
  dCl(alpha,aileron) : Interpolation_n-D  Table=dCroll_aileron
  dCl(alpha,beta) : Interpolation_n-D  Table=Croll_datum
  dCl(alpha,rudder) : Interpolation_n-D  Table=dCroll_rudder
  rudder_interp : PreLookup  BreakpointsData=rudder  BeginIndexSearchUsingPreviousIndexResult=on  ExtrapMethod=Linear
  Net Cl : Outport  VectorParamsAs1DForOutWhenUnconnected=off
  wires:
  beta (deg)/1 -> beta_interp/1
  Sum/1 -> Scope/1, Net Cl/1
  aileron (deg)/1 -> aileron_interp/1
  rudder (deg)/1 -> rudder_interp/1
  beta_interp/1 -> dCl(alpha,beta)/3
  beta_interp/2 -> dCl(alpha,beta)/4
  rudder_interp/2 -> dCl(alpha,rudder)/4
  aileron_interp/1 -> dCl(alpha,aileron)/3
  aileron_interp/2 -> dCl(alpha,aileron)/4
  rudder_interp/1 -> dCl(alpha,rudder)/3
  alpha (deg)/1 -> alpha_interp1/1, alpha_interp/1
  alpha_interp/2 -> dCl(alpha,rudder)/2, dCl(alpha,beta)/2
  alpha_interp/1 -> dCl(alpha,rudder)/1, dCl(alpha,beta)/1
  dCl(alpha,aileron)/1 -> Sum/2
  dCl(alpha,rudder)/1 -> Sum/3
  dCl(alpha,beta)/1 -> Sum/1
  alpha_interp1/1 -> dCl(alpha,aileron)/1
  alpha_interp1/2 -> dCl(alpha,aileron)/2

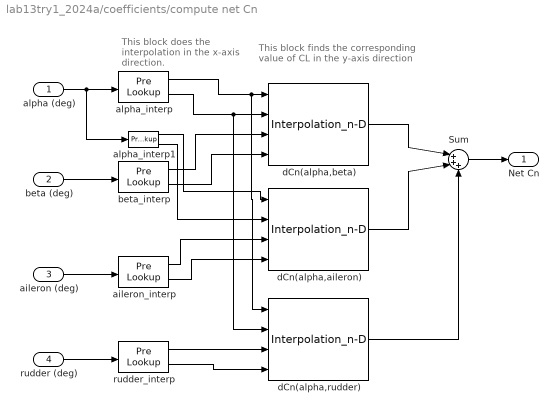
== system lab13try1_2024a/coefficients/compute net Cn ==
  note: This block finds the corresponding
      | value of CL in the y-axis direction
  note: This block does the interpolation in the
      | x-axis direction.
  alpha (deg) : Inport
  beta (deg) : Inport  Port=2
  aileron (deg) : Inport  Port=3
  rudder (deg) : Inport  Port=4
  Sum : Sum  Inputs=|+++
  aileron_interp : PreLookup  BreakpointsData=aileron  BeginIndexSearchUsingPreviousIndexResult=on  ExtrapMethod=Linear
  alpha_interp : PreLookup  BreakpointsData=alphalatrud  BeginIndexSearchUsingPreviousIndexResult=on  ExtrapMethod=Linear
  alpha_interp1 : PreLookup  BreakpointsData=alphaaileron  BeginIndexSearchUsingPreviousIndexResult=on  ExtrapMethod=Linear
  beta_interp : PreLookup  BreakpointsData=beta  BeginIndexSearchUsingPreviousIndexResult=on  ExtrapMethod=Linear
  dCn(alpha,aileron) : Interpolation_n-D  Table=dCn_aileron
  dCn(alpha,beta) : Interpolation_n-D  Table=Cn_datum
  dCn(alpha,rudder) : Interpolation_n-D  Table=dCn_rudder
  rudder_interp : PreLookup  BreakpointsData=rudder  BeginIndexSearchUsingPreviousIndexResult=on  ExtrapMethod=Linear
  Net Cn : Outport  VectorParamsAs1DForOutWhenUnconnected=off
  wires:
  beta (deg)/1 -> beta_interp/1
  Sum/1 -> Net Cn/1
  aileron (deg)/1 -> aileron_interp/1
  rudder (deg)/1 -> rudder_interp/1
  beta_interp/1 -> dCn(alpha,beta)/3
  beta_interp/2 -> dCn(alpha,beta)/4
  rudder_interp/2 -> dCn(alpha,rudder)/4
  aileron_interp/1 -> dCn(alpha,aileron)/3
  aileron_interp/2 -> dCn(alpha,aileron)/4
  rudder_interp/1 -> dCn(alpha,rudder)/3
  alpha (deg)/1 -> alpha_interp1/1, alpha_interp/1
  alpha_interp/2 -> dCn(alpha,rudder)/2, dCn(alpha,beta)/2
  alpha_interp/1 -> dCn(alpha,rudder)/1, dCn(alpha,beta)/1
  dCn(alpha,beta)/1 -> Sum/1
  dCn(alpha,aileron)/1 -> Sum/2
  dCn(alpha,rudder)/1 -> Sum/3
  alpha_interp1/1 -> dCn(alpha,aileron)/1
  alpha_interp1/2 -> dCn(alpha,aileron)/2
